simulink model "Question8Hw1Sim_AkankshaMurali"  (R2023b)
settings: Solver=VariableStepAuto  StartTime=0.0  StopTime=10.0  RelTol=1e-3
settings Model: Creator=shash  LastModifiedBy=akank

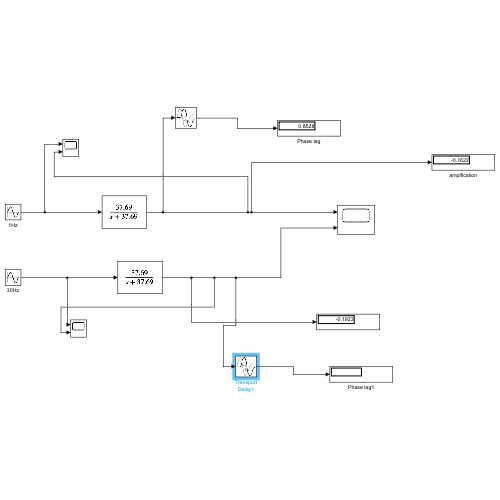
[thumbnail: Simulink's stored preview of the top-level diagram]
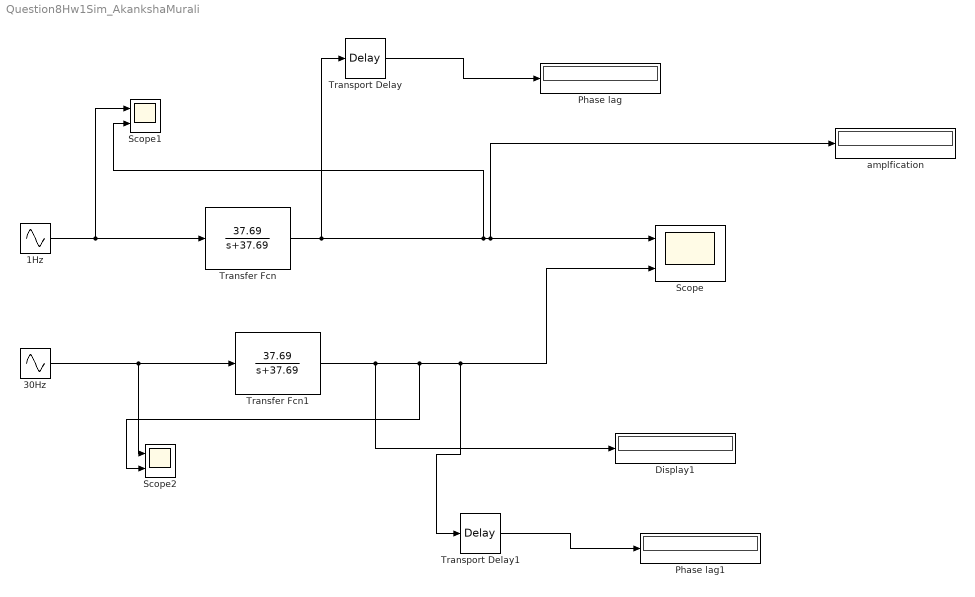
== system Question8Hw1Sim_AkankshaMurali ==
  1Hz : Sin  Frequency=6.2831853  SampleTime=0
  30Hz : Sin  Frequency=188.495559  SampleTime=0
  Display1 : Display
  Phase lag : Display
  Phase lag1 : Display
  Scope : Scope  NumInputPorts=2
  Scope1 : Scope  NumInputPorts=2
  Scope2 : Scope  NumInputPorts=2
  Transfer Fcn : TransferFcn  Numerator=[37.69]  Denominator=[1 37.69]
  Transfer Fcn1 : TransferFcn  Numerator=[37.69]  Denominator=[1 37.69]
  Transport Delay : TransportDelay  DelayTime=0.64
  Transport Delay1 : TransportDelay  DelayTime=0.00762
  amplfication : Display
  wires:
  30Hz/1 -> Scope2/1, Transfer Fcn1/1
  Transfer Fcn1/1 -> Display1/1, Scope2/2, Transport Delay1/1, Scope/2
  Transfer Fcn/1 -> Scope1/2, amplfication/1, Scope/1, Transport Delay/1
  1Hz/1 -> Scope1/1, Transfer Fcn/1
  Transport Delay/1 -> Phase lag/1
  Transport Delay1/1 -> Phase lag1/1
